simulink model "darko_control_lineaire_vol_virage"  (R2020b)
settings: Solver=VariableStepAuto  StartTime=0.0  StopTime=20  RelTol=1e-3
values from neighbouring files (symbols this model uses):
  drone = generateDarko()    [main_linearisation_vol_virage.m]
  initial_state = x_eq    [main_linearisation_vol_virage.m]
  K_lin_control = [zeros(4,2), K_lin(:,1:4), zeros(4,4), K_lin(:,5:7)]    [main_linearisation_vol_virage.m]
  u_eq = [trim(1); trim(1); trim(2); trim(2)]    [main_linearisation_vol_virage.m]
  x_eq = [p_initial; v_initial; q_initial; omega_initial]    [main_linearisation_vol_virage.m]
undefined symbols (not defined in the file or in its folder): S_complet
libraries: simulink_extras x3, sharedtransform x1, simulink x1
settings Model: Creator=florian  LastModifiedBy=florian

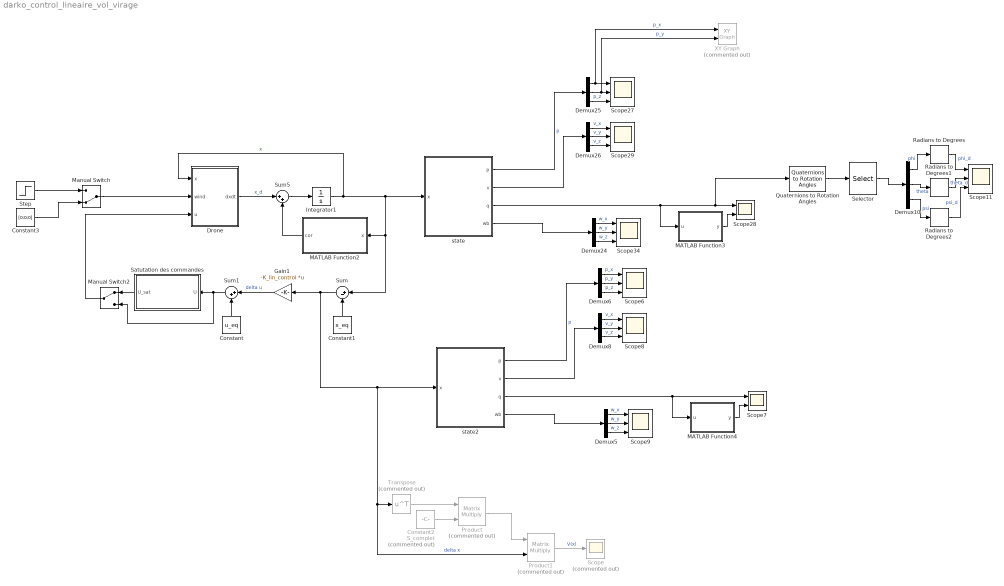
== system darko_control_lineaire_vol_virage ==
  Constant : Constant  Value=u_eq
  Constant1 : Constant  Value=x_eq
  Constant2 : Constant  Commented=on  Value=S_complet
  Constant3 : Constant  Value=[0;0;0]
  Demux{5..6,8,10,24..26} (7 alike) : Demux  Outputs=3
  Drone : MATLAB Function  TreatAsAtomicUnit=on
  Gain1 : Gain  Gain=-K_lin_control  Multiplication=Matrix(K*u) (u vector)
  Integrator1 : Integrator  InitialCondition=initial_state
  MATLAB Function2 : MATLAB Function  TreatAsAtomicUnit=on
  MATLAB Function3 : MATLAB Function  TreatAsAtomicUnit=on
  MATLAB Function4 : MATLAB Function  TreatAsAtomicUnit=on
  Manual Switch : ManualSwitch  CurrentSetting=0
  Manual Switch2 : ManualSwitch
  Product : Product  Commented=on  Multiplication=Matrix(*)
  Product1 : Product  Commented=on  Multiplication=Matrix(*)
  Quaternions to Rotation Angles : sharedtransform/Quaternions to Rotation Angles  rotationOrder=ZXY  aMode=aMode
      settings: SourceProductBaseCode=AE,PW,MT,UV,VE,VP
  Radians to Degrees : simulink_extras/Transformations/Radians to Degrees
  Radians to Degrees1 : simulink_extras/Transformations/Radians to Degrees
  Radians to Degrees2 : simulink_extras/Transformations/Radians to Degrees
  Satutation des commandes : Subsystem
  Scope : Scope  Commented=on
  Scope{6,8..9,11,27,29,34} (7 alike) : Scope  NumInputPorts=3
  Scope28 : Scope  NumInputPorts=2
  Scope7 : Scope  NumInputPorts=2
  Selector : Selector  InputPortWidth=3  IndexOptions=Index vector (dialog)  Indices=[2 3 1]  OutputSizes=1
  Step : Step  Time=10  Before=[0;0;0]  After=[-5;0;0]  SampleTime=0
  Sum : Sum  Inputs=|+-
  Sum1 : Sum  Inputs=|++
  Sum5 : Sum  Inputs=|++
  Transpose : Math  Commented=on  Operator=transpose  SaturateOnIntegerOverflow=on
  XY Graph : simulink/Sinks/XY Graph  Commented=on  xmin=0  xmax=100  ymin=-100  ymax=0  st=-1
  state : MATLAB Function  TreatAsAtomicUnit=on
  state2 : MATLAB Function  TreatAsAtomicUnit=on
  wires:
  Sum5/1 -> Integrator1/1
  MATLAB Function2/1(cor) -> Sum5/2
  Drone/1(dxdt) -> Sum5/1  "x_d"
  Demux25/3 -> Scope27/3  "p_z"
  Demux26/2 -> Scope29/2  "v_y"
  Demux24/1 -> Scope34/1  "w_x"
  MATLAB Function3/1(y) -> Scope28/2
  state/3(q) -> MATLAB Function3/1(u), Quaternions to Rotation Angles/1, Scope28/1
  Demux25/1 -> XY Graph/1, Scope27/1  "p_x"
  state/4(wb) -> Demux24/1
  Demux24/2 -> Scope34/2  "w_y"
  state/1(p) -> Demux25/1  "p"
  Demux24/3 -> Scope34/3  "w_z"
  state/2(v) -> Demux26/1
  Demux25/2 -> XY Graph/2, Scope27/2  "p_y"
  Demux26/3 -> Scope29/3  "v_z"
  Demux26/1 -> Scope29/1  "v_x"
  Sum/1 -> Product1/2, Transpose/1, state2/1(x), Gain1/1  "delta x"
  Gain1/1 -> Sum1/1  "delta u"
  Constant/1 -> Sum1/2
  Constant1/1 -> Sum/2
  Demux6/3 -> Scope6/3  "p_z"
  Demux8/2 -> Scope8/2  "v_y"
  state2/3(q) -> MATLAB Function4/1(u), Scope7/1
  state2/4(wb) -> Demux5/1
  MATLAB Function4/1(y) -> Scope7/2
  Demux5/2 -> Scope9/2  "w_y"
  Demux8/3 -> Scope8/3  "v_z"
  Demux6/1 -> Scope6/1  "p_x"
  Demux5/1 -> Scope9/1  "w_x"
  Demux8/1 -> Scope8/1  "v_x"
  state2/1(p) -> Demux6/1  "p"
  Demux6/2 -> Scope6/2  "p_y"
  Demux5/3 -> Scope9/3  "w_z"
  state2/2(v) -> Demux8/1
  Product1/1 -> Scope/1  "V(x)"
  Transpose/1 -> Product/1
  Constant2/1 -> Product/2
  Product/1 -> Product1/1
  Manual Switch/1 -> Drone/2(wind)
  Step/1 -> Manual Switch/1
  Constant3/1 -> Manual Switch/2
  Demux10/2 -> Radians to Degrees1/1  "theta"
  Demux10/1 -> Radians to Degrees/1  "phi"
  Radians to Degrees1/1 -> Scope11/2  "theta_d"
  Demux10/3 -> Radians to Degrees2/1  "psi"
  Radians to Degrees/1 -> Scope11/1  "phi_d"
  Quaternions to Rotation Angles/1 -> Selector/1
  Radians to Degrees2/1 -> Scope11/3  "psi_d"
  Selector/1 -> Demux10/1
  Integrator1/1 -> Drone/1(x), state/1(x), Sum/1, MATLAB Function2/1(x)  "x"
  Satutation des commandes/1(U_sat) -> Manual Switch2/1
  Manual Switch2/1 -> Drone/3(u)
  Sum1/1 -> Manual Switch2/2, Satutation des commandes/1(U)

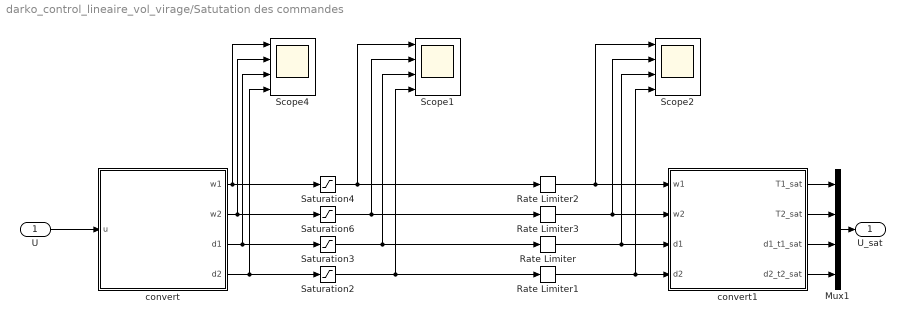
== system darko_control_lineaire_vol_virage/Satutation des commandes ==
  U : Inport
  Mux1 : Mux
  Rate Limiter : RateLimiter  RisingSlewLimit=drone.ELEVON_RATE_CHANGE  FallingSlewLimit=-drone.ELEVON_RATE_CHANGE  SampleTimeMode=inherited
  Rate Limiter1 : RateLimiter  RisingSlewLimit=drone.ELEVON_RATE_CHANGE  FallingSlewLimit=-drone.ELEVON_RATE_CHANGE  SampleTimeMode=inherited
  Rate Limiter2 : RateLimiter  RisingSlewLimit=drone.MOTOR_RATE_CHANGE  FallingSlewLimit=-drone.MOTOR_RATE_CHANGE  SampleTimeMode=inherited
  Rate Limiter3 : RateLimiter  RisingSlewLimit=drone.MOTOR_RATE_CHANGE  FallingSlewLimit=-drone.MOTOR_RATE_CHANGE  SampleTimeMode=inherited
  Saturation2 : Saturate  UpperLimit=30*(pi/180)  LowerLimit=-30*(pi/180)
  Saturation3 : Saturate  UpperLimit=30*(pi/180)  LowerLimit=-30*(pi/180)
  Saturation4 : Saturate  UpperLimit=1000  LowerLimit=200
  Saturation6 : Saturate  UpperLimit=1000  LowerLimit=200
  Scope1 : Scope  NumInputPorts=4
  Scope2 : Scope  NumInputPorts=4
  Scope4 : Scope  NumInputPorts=4
  convert : MATLAB Function  TreatAsAtomicUnit=on
  convert1 : MATLAB Function  TreatAsAtomicUnit=on
  U_sat : Outport
  wires:
  U/1 -> convert/1(u)
  convert/1(w1) -> Saturation4/1, Scope4/1
  Saturation3/1 -> Rate Limiter/1, Scope1/3
  convert/2(w2) -> Scope4/2, Saturation6/1
  convert/3(d1) -> Scope4/3, Saturation3/1
  convert/4(d2) -> Saturation2/1, Scope4/4
  convert1/1(T1_sat) -> Mux1/1
  convert1/4(d2_t2_sat) -> Mux1/4
  Mux1/1 -> U_sat/1
  convert1/2(T2_sat) -> Mux1/2
  convert1/3(d1_t1_sat) -> Mux1/3
  Saturation2/1 -> Rate Limiter1/1, Scope1/4
  Rate Limiter/1 -> Scope2/3, convert1/3(d1)
  Saturation6/1 -> Rate Limiter3/1, Scope1/2
  Saturation4/1 -> Rate Limiter2/1, Scope1/1
  Rate Limiter1/1 -> Scope2/4, convert1/4(d2)
  Rate Limiter2/1 -> Scope2/1, convert1/1(w1)
  Rate Limiter3/1 -> Scope2/2, convert1/2(w2)

== matlab function darko_control_lineaire_vol_virage/Drone ==
  data: x input; wind input; u input; dxdt output; drone parameter
function dxdt  = drone(x,wind, u, drone)

%% physical constants
% gravity
g = drone.G;
% vehicle mass
m = drone.MASS;
% vehicle inertia matrix
J = drone.INERTIA; % [3x3 real symmetric] in body axis

%% state demultiplexing
% p = x(1:3);
v = x(4:6);
q  = x(7:10);
wb = x(11:13);

Rq = q2dcm(q);

[Fp, Mp] = external_force_moment(x, u, wind, drone);

% position
dpdt = v;

% kinematics
dvdt =  -[0;0;g] + (1/m)*Rq*drone.Fb*u + (1/m)*Rq*Fp; 

%% quaternion derivative
eta = q(1);
eps = q(2:4);

dqdt = (1/2)*[-eps'; eta*eye(3) + skew_sym(eps)]*wb;

%% angular velocity derivative
% kinematics
dwdt = -J\cross(wb, J*wb) + J\(drone.Mb*u) + J\Mp;


%% derivative multiplexing
dxdt = [dpdt; dvdt; dqdt; dwdt] ;

== matlab function darko_control_lineaire_vol_virage/MATLAB Function4 ==
  data: u input; y output
function y = fcn(u)
%#codegen

y = norm(u);

== matlab function darko_control_lineaire_vol_virage/state2 ==
  data: x input; p output; v output; q output; wb output
function [p, v, q, wb] = demux(x)
%#codegen

p = x(1:3);
v = x(4:6);
q  = x(7:10);
wb = x(11:13);

== matlab function darko_control_lineaire_vol_virage/Satutation des commandes/convert ==
  data: u input; w1 output; drone parameter; w2 output; d1 output; d2 output
function [w1, w2, d1, d2] = convert(u, drone)
%#codegen
kf = drone.PROP_KP;

T1 = max(u(1),0);
T2 = max(u(1),0);
d1_T1 = u(3);
d2_T2 = u(4);

w1 = sqrt(T1/kf);
w2 = sqrt(T2/kf);
d1 = d1_T1/T1;
d2 = d2_T2/T2;

== matlab function darko_control_lineaire_vol_virage/Satutation des commandes/convert1 ==
  data: w1 input; w2 input; d1 input; d2 input; T1_sat output; T2_sat output; drone parameter; d1_t1_sat output; d2_t2_sat output
function [T1_sat, T2_sat, d1_t1_sat, d2_t2_sat] = convert2(w1, w2, d1, d2, drone)
%#codegen
kf = drone.PROP_KP;

T1_sat = kf*w1^2;
d1_t1_sat = d1*T1_sat;
T2_sat = kf*w2^2;
d2_t2_sat = d2*T2_sat;

== matlab function darko_control_lineaire_vol_virage/MATLAB Function2 ==
  data: x input; cor output
function cor  = fcn(x)
%#codegen
q  = x(7:10);
n = norm(q);
mismatch = 1-n;
cor = [0;0;0; 0;0;0; mismatch*q; 0;0;0];

== matlab function darko_control_lineaire_vol_virage/MATLAB Function3 ==
  data: u input; y output
function y = fcn(u)
%#codegen

y = norm(u);

== matlab function darko_control_lineaire_vol_virage/state ==
  data: x input; p output; v output; q output; wb output
function [p, v, q, wb] = demux(x)
%#codegen

p = x(1:3);
v = x(4:6);
q  = x(7:10);
wb = x(11:13);
